simulink model "experiments_swing_up_energy"  (R2019b)
settings: Solver=ode1  StartTime=0.0  StopTime=inf  FixedStep=0.002  RelTol=1e-3  EnableMultiTasking=on
PostLoadFcn:
  | qc_set_target_type(getConfigSet(bdroot, 'QUARC Default Target Configuration'));
undefined symbols (not defined in the file): HIL, Klqi_state, Parameters, qc_get_step_size
libraries: quarc_library x4
settings Model: SimulationMode=external  ExtModeTrigDuration=5000  Creator=CFulford  LastModifiedBy=Student
settings SolverCC: PositivePriorityOrder=on
settings DataIOCC: LimitDataPoints=on  SaveFormat=Array  SignalLoggingSaveFormat=ModelDataLogs  ReturnWorkspaceOutputs=off
settings OptimizationCC: ExpressionDepthLimit=2147483647  InitFltsAndDblsToZero=on  LifeSpan=inf
settings DebuggingCC: SaveWithParameterizedLinksMsg=none  UnderspecifiedInitializationDetection=Classic  MergeDetectMultiDrivingBlocksExec=none  SolverPrmCheckMsg=warning  MultiTaskDSMMsg=warning  MultiTaskCondExecSysMsg=none  FcnCallInpInsideContextMsg=warning  StateNameClashWarn=warning  SFUnexpectedBacktrackingDiag=warning  SFNoUnconditionalDefaultTransitionDiag=warning  SFExecutionAtInitializationDiag=none  ArithmeticOperatorsInVariantConditions=warning
settings HardwareCC: ProdBitPerPointer=32  ProdBitPerSizeT=32  ProdBitPerPtrDiffT=32  ProdLargestAtomicFloat=None  ProdIntDivRoundTo=Undefined  ProdEndianess=Unspecified  ProdWordSize=32  ProdHWDeviceType=32-bit Generic
settings ModelReferenceCC: PropagateSignalLabelsOutOfModel=off
settings SFSimCC: SimUseLocalCustomCode=off  CustomCodeUndefinedFunction=UseInterfaceOnly
settings RTWCC: Description=QUARC Win64 Target  SystemTargetFile=quarc_win64.tlc  TemplateMakefile=quarc_default_tmf  RTWUseLocalCustomCode=off
settings CodeAppCC: StateflowObjectComments=on
settings STFCustomTargetCC: TargetPreCompLibLocation=C:\PROGRA~3\QUARC\lib\2019b\win64\release  ConcurrentExecutionCompliant=on  GeneratePreprocessorConditionals=Disable all  CombineOutputUpdateFcns=on  CPPClassGenCompliant=on  SystemTargetFile=quarc_win64.tlc
settings GRTTargetCC: TargetPreCompLibLocation=C:\PROGRA~3\QUARC\lib\2019b\win64\release  TargetLangStandard=C89/C90 (ANSI)  ParMdlRefBuildCompliant=off  CompOptLevelCompliant=off  GeneratePreprocessorConditionals=Disable all  MatFileLogging=off  UseToolchainInfoCompliant=off  ExtMode=on  ExtModeMexFile=quarc_comm
settings ConfigComp: CovMetricSettings=dw  CovHtmlReporting=on  CovSaveCumulativeToWorkspaceVar=on  CovSaveSingleToWorkspaceVar=on  CovExternalEMLEnable=off  CovSFcnEnable=off

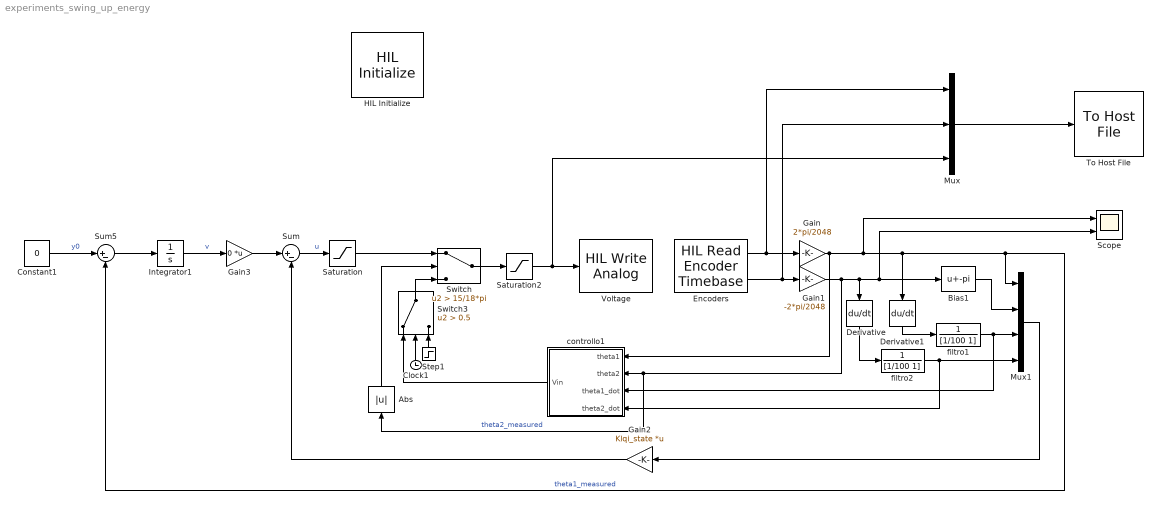
== system experiments_swing_up_energy ==
  Abs : Abs
  Bias1 : Bias  Bias=-pi
  Clock1 : Clock
  Constant1 : Constant  Value=0
  Derivative : Derivative
  Derivative1 : Derivative
  Encoders : quarc_library/Data Acquisition/Generic/Timebases/HIL Read Encoder Timebase  object_name=HIL-1  clock=0  channels=[0:1]  samples_in_buffer=max(ceil(1/qc_get_step_size), 1)  active=on  vector_output=off  data_type_mode=Inherit via back propagation  data_type=double
  Gain : Gain  Gain=2*pi/2048
  Gain1 : Gain  Gain=-2*pi/2048
  Gain2 : Gain  Gain=Klqi_state  Multiplication=Matrix(K*u)
  Gain3 : Gain  Gain=0  Multiplication=Matrix(K*u)
  HIL Initialize : quarc_library/Data Acquisition/Generic/Configuration/HIL Initialize  Priority=-99  object_name=HIL-1  board_type=qube_servo2_usb  board_number=0  board_options=""  exclusive=off  active=off  hardware_clocks=[0]  clock_modes=[]  initial_clock_frequencies=[]  set_clock_params_at_start=off  set_clock_params_at_switch_in=off  set_clock_frequencies_at_start=off  set_clock_frequencies_at_switch_in=off  analog_input_channels=[0]  analog_input_configurations=[]  analog_input_maximums=3  analog_input_minimums=-3  set_analog_input_params_at_start=off  set_analog_input_params_at_switch_in=off  analog_output_channels=[0]  analog_output_maximums=15  analog_output_minimums=-15  initial_analog_outputs=[0]  final_analog_outputs=[0]  watchdog_analog_outputs=0  set_analog_output_params_at_start=off  set_analog_output_params_at_switch_in=off  set_analog_outputs_at_start=on  set_analog_outputs_at_switch_in=off  set_analog_outputs_at_terminate=on  set_analog_outputs_at_switch_out=off  set_analog_outputs_on_watchdog=on  digital_input_channels=[]  digital_output_channels=[0]  digital_output_configuration=[]  initial_digital_outputs=[1]  final_digital_outputs=[0]  watchdog_digital_outputs=[0]  set_digital_output_params_at_start=off  set_digital_output_params_at_switch_in=off  set_digital_outputs_at_start=on  set_digital_outputs_at_switch_in=off  set_digital_outputs_at_terminate=on  set_digital_outputs_at_switch_out=off  set_digital_outputs_on_watchdog=on  encoder_channels=[0:1]  quadrature=[4]  encoder_filter_frequency=[]  initial_encoder_counts=[0]  set_encoder_params_at_start=off  set_encoder_params_at_switch_in=off  set_encoder_counts_at_start=on  set_encoder_counts_at_switch_in=off  pwm_channels=[]  pwm_modes=[]  pwm_frequency=[]  pwm_configuration=[]  pwm_alignment=[]  pwm_polarity=[]  pwm_leading_deadband=[]  pwm_trailing_deadband=[]  initial_pwm_outputs=[]  final_pwm_outputs=[]  watchdog_pwm_outputs=[]  set_pwm_params_at_start=off  set_pwm_params_at_switch_in=off  set_pwm_outputs_at_start=off  set_pwm_outputs_at_switch_in=off  set_pwm_outputs_at_terminate=off  set_pwm_outputs_at_switch_out=off  set_pwm_outputs_on_watchdog=off  other_output_channels=[11000:11002]  initial_other_outputs=[0 1 0]  final_other_outputs=[1 0 0]  watchdog_other_outputs=[0 0 1]  set_other_outputs_at_start=on  set_other_outputs_at_switch_in=off  set_other_outputs_at_terminate=on  set_other_outputs_at_switch_out=off  set_other_outputs_on_watchdog=on
  Integrator1 : Integrator
  Mux : Mux  Inputs=3
  Mux1 : Mux
  Saturation : Saturate  UpperLimit=10  LowerLimit=-10
  Saturation2 : Saturate  UpperLimit=10  LowerLimit=-10  ZeroCross=off
  Scope : Scope  NumInputPorts=2
  Step1 : Step  Time=0.1  After=-1  SampleTime=0
  Sum : Sum  Inputs=|+-
  Sum5 : Sum  Inputs=|+-
  Switch : Switch  Criteria=u2 > Threshold  Threshold=15/18*pi
  Switch3 : Switch  Criteria=u2 > Threshold  Threshold=0.5
  To Host File : quarc_library/Sinks/To Host/To Host File  file_name=data_%{date}_%{time}.mat  variable_name=data_%{date}_%{time}  decimation=1  sample_time=-1  file_format=MAT-file v.5  options=No header or footer  append=off  final_file_name=data_28-May-2024_15-43-59.mat  bitrate=2000000
  Voltage : quarc_library/Data Acquisition/Generic/Immediate I//O/HIL Write Analog  object_name=HIL-1  channels=0  sample_time=-1  active=off  vector_input=off
  controllo1 : Subsystem
  "filtro1 " : TransferFcn  Denominator=[1/100 1]
  filtro2 : TransferFcn  Denominator=[1/100 1]
  wires:
  Mux/1 -> To Host File/1
  Gain2/1 -> Sum/2
  Encoders/2 -> Mux/2, Gain1/1
  Switch/1 -> Saturation2/1
  Mux1/1 -> Gain2/1
  "filtro1 "/1 -> controllo1/3(theta1_dot), Mux1/3
  Gain3/1 -> Sum/1
  Derivative/1 -> filtro2/1
  Derivative1/1 -> "filtro1 "/1
  Encoders/1 -> Mux/1, Gain/1
  Sum/1 -> Saturation/1  "u"
  Integrator1/1 -> Gain3/1  "v"
  filtro2/1 -> controllo1/4(theta2_dot), Mux1/4
  Gain/1 -> Scope/1, Sum5/2, Mux1/1, Derivative1/1, controllo1/1(theta1)  "theta1_measured"
  Sum5/1 -> Integrator1/1
  Saturation/1 -> Switch/1
  Gain1/1 -> Scope/2, Bias1/1, Derivative/1, Abs/1, controllo1/2(theta2)  "theta2_measured"
  Constant1/1 -> Sum5/1  "y0"
  Abs/1 -> Switch/2
  Bias1/1 -> Mux1/2
  Step1/1 -> Switch3/3
  Clock1/1 -> Switch3/2
  Switch3/1 -> Switch/3
  controllo1/1(Vin) -> Switch3/1
  Saturation2/1 -> Mux/3, Voltage/1

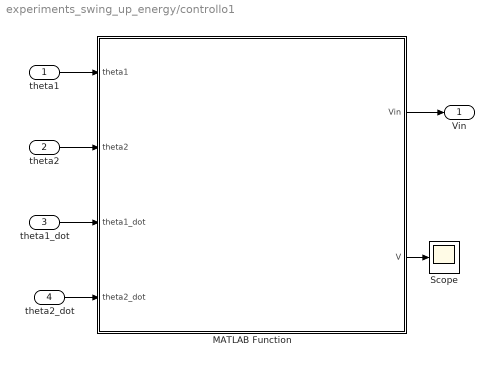
== system experiments_swing_up_energy/controllo1 ==
  theta1 : Inport
  theta2 : Inport  Port=2
  theta1_dot : Inport  Port=3
  theta2_dot : Inport  Port=4
  MATLAB Function : MATLAB Function  TreatAsAtomicUnit=on  mask{Pars=Parameters}
      mask prompts: Pars "Struct containing model parameters"
  Scope : Scope
  Vin : Outport
  wires:
  MATLAB Function/1(Vin) -> Vin/1
  theta1/1 -> MATLAB Function/1(theta1)
  theta2/1 -> MATLAB Function/2(theta2)
  theta1_dot/1 -> MATLAB Function/3(theta1_dot)
  theta2_dot/1 -> MATLAB Function/4(theta2_dot)
  MATLAB Function/2(V) -> Scope/1

== matlab function experiments_swing_up_energy/controllo1/MATLAB Function ==
  data: theta1 input size=1; Vin output size=1; theta2 input size=1; theta1_dot input size=1; theta2_dot input size=1; Pars parameter; V output
function [Vin, V]  = fcn(theta1, theta2, theta1_dot, theta2_dot, Pars)
   const = 1000*0.9;
   k1 = Pars.Jeq + Pars.m2*(Pars.l1^2 + Pars.x2^2*sin(theta2)^2);
   k2 = Pars.m2*Pars.l1*Pars.x2*cos(theta2);
   % attenzione k3 diverso da funzione modello non lineare 
   k3 = 2*Pars.m2*Pars.x2^2*sin(theta2)*cos(theta2)*theta1_dot*theta2_dot - Pars.m2*Pars.l1*Pars.x2*sin(theta2)*theta2_dot^2 +Pars.Ks*theta1 + (Pars.Km^2)/Pars.Rm*theta1_dot + Pars.Kf1*theta1_dot;
   k4 = Pars.m2*Pars.l1*Pars.x2*cos(theta2);
   k5 = Pars.m2*Pars.x2^2 + Pars.I2;
   k6 = - Pars.m2*Pars.x2^2*sin(theta2)*cos(theta2)*theta1_dot^2 + Pars.m2*Pars.g*Pars.x2*sin(theta2) + Pars.Kf2*theta2_dot;
   
   % energia = energia cinetica + energia potenziale (prendo come 0 down)
   E = 1/2*(Pars.I2+Pars.m2*Pars.x2^2)*theta2_dot^2 + Pars.m2*Pars.g*(Pars.x2-Pars.x2*cos(theta2));
   Eup = Pars.m2*Pars.g*(Pars.x2+Pars.x2)*1.1; %aumento un po' Eup per attrito
   
   % funzione di Lyapunov V>0
   V = 1/2*(E-Eup)^2;
   
   % derivata lyapunov Vdot
   %Vdot = (E-Eup)*theta2_dot*((Pars.I2+Pars.m2*Pars.x2^2)*theta2_dot_dot+Pars.m2*Pars.g*Pars.x2*sin(theta2));
   
   % impongo theta2dotdot tale che derivata di V <0
   theta2_dot_dot = -Pars.m2*Pars.g*Pars.x2*sin(theta2)/(Pars.I2+Pars.m2*Pars.x2^2) -const*(E-Eup)*sign(theta2_dot);
   
   % calcolo Vin in base a modello non lineare
   Vin = (k4*k3-k1*k6-theta2_dot_dot*(k1*k5-k2*k4))*Pars.Rm/Pars.Km/k4;
   
end
